simulink model "PieroModel"  (R2023b)
settings: Solver=VariableStepAuto  StartTime=0.0  StopTime=10.0  RelTol=1e-3
settings Model: Creator=Daniel  LastModifiedBy=Daniel

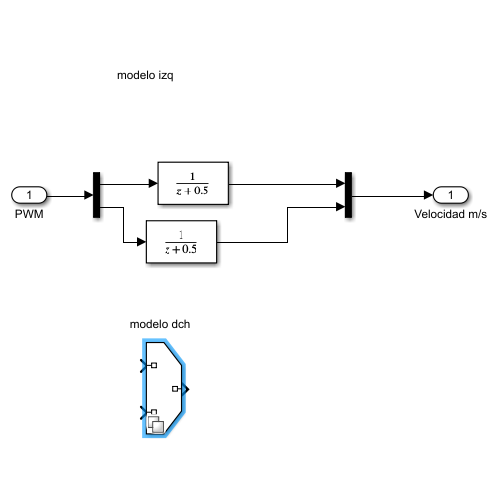
[thumbnail: Simulink's stored preview of the top-level diagram]
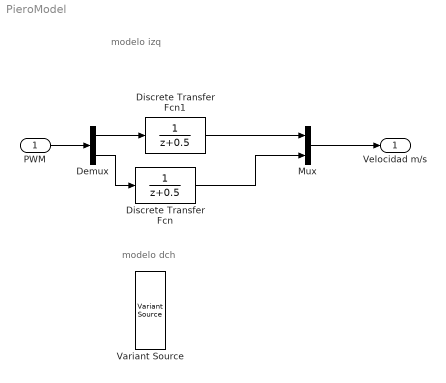
== system PieroModel ==
  note: modelo dch
  note: modelo izq
  PWM : Inport
  Demux : Demux  Outputs=2
  Discrete Transfer Fcn : DiscreteTransferFcn
  Discrete Transfer Fcn1 : DiscreteTransferFcn
  Mux : Mux  Inputs=2
  Variant Source : VariantSource
  Velocidad m/s : Outport
  wires:
  PWM/1 -> Demux/1
  Mux/1 -> Velocidad m/s/1
  Demux/1 -> Discrete Transfer Fcn1/1
  Discrete Transfer Fcn1/1 -> Mux/1
  Demux/2 -> Discrete Transfer Fcn/1
  Discrete Transfer Fcn/1 -> Mux/2
